simulink subsystem "PowerGain"  (R2023a)
settings: Solver=VariableStepAuto  StartTime=0.0  StopTime=10.0  RelTol=1e-3
model mask{Ku=27/3.3, up_lim=24, low_lim=0}
  mask prompts: Ku "gain factor"; up_lim "upper limit"; low_lim "lower limit"
settings Model: Creator=ASUS TUF GAMING  LastModifiedBy=ASUS TUF GAMING

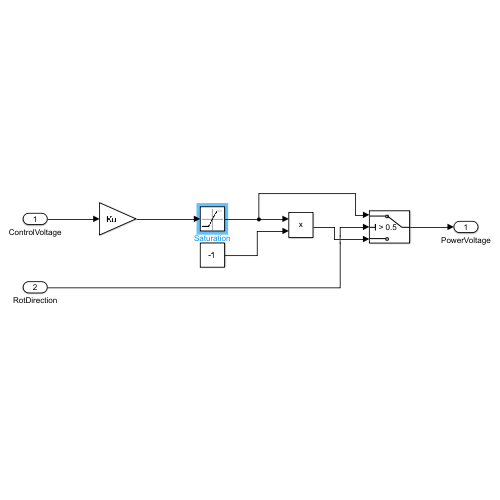
[thumbnail: Simulink's stored preview of the top-level diagram]
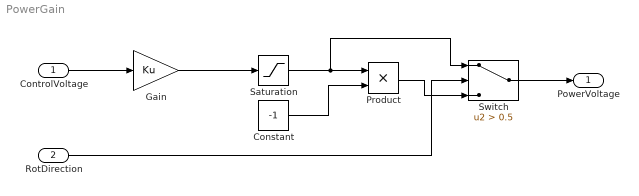
== system PowerGain ==
  ControlVoltage : Inport
  RotDirection : Inport  Port=2
  Constant : Constant  Value=-1
  Gain : Gain  Gain=Ku
  Product : Product
  Saturation : Saturate  UpperLimit=up_lim  LowerLimit=low_lim
  Switch : Switch  Criteria=u2 > Threshold  Threshold=0.5  SaturateOnIntegerOverflow=off  InputSameDT=off
  PowerVoltage : Outport
  wires:
  ControlVoltage/1 -> Gain/1
  Gain/1 -> Saturation/1
  Saturation/1 -> Switch/1, Product/1
  Constant/1 -> Product/2
  Product/1 -> Switch/3
  RotDirection/1 -> Switch/2
  Switch/1 -> PowerVoltage/1
